simulink model "ASLIPrun2_returnmap"  (R2016a)
settings: Solver=ode45  StartTime=0.0  StopTime=250  MaxStep=1e-3  RelTol=1e-4  AbsTol=1e-6
values from neighbouring files (symbols this model uses):
  a0 = 67*pi/180    (= 1.16937059884)    [ASLIPrun_params2.m]
  dt0 = deg2rad(0)    [ASLIPrun_params2.m]
  dx0 = 5.00    (= 5)    [ASLIPrun_params2.m]
  dy0 = 0    [ASLIPrun_params2.m]
  g = 9.81    [ASLIPrun_params2.m]
  J = 4.58    [ASLIPrun_params2.m]
  k = 20000    [ASLIPrun_params2.m]
  kt = 100    [ASLIPrun_params2.m]
  L = 0.1    [ASLIPrun_params2.m]    (also in AnimSMR2.m = sqrt( (u(4)-u(9))^2 + (u(5)-u(10))^2 ))
  l0 = 1    [ASLIPrun_params2.m]
  m = 80    [ASLIPrun_params2.m]
  model = 1    [ASLIPrun_params2.m]
  r0 = sqrt(xr0^2 + yr0^2)    [ASLIPrun_params2.m]
  rp = 0.005    [ASLIPrun_params2.m]
  t0 = 70*pi/180    (= 1.2217304764)    [ASLIPrun_params2.m]
  x0 = 0*(-l0 + L*cos(t0))    [ASLIPrun_params2.m]    (also in AnimSMR2.m = [])
  xr0 = -l0*cos(a0) + L*cos(t0)    [ASLIPrun_params2.m]
  y0 = 1.065    [ASLIPrun_params2.m]
  yr0 = l0*sin(a0) + L*sin(t0)    [ASLIPrun_params2.m]
libraries: simulink_extras x1
settings Model: Creator=hgeyer  LastModifiedBy=Joe
settings DataIOCC: SaveFormat=Array  SignalLoggingSaveFormat=ModelDataLogs
settings OptimizationCC: ExpressionDepthLimit=2147483647
settings DebuggingCC: UnderspecifiedInitializationDetection=Classic  MergeDetectMultiDrivingBlocksExec=none  SolverPrmCheckMsg=warning  FcnCallInpInsideContextMsg=EnableAllAsWarning  StateNameClashWarn=warning
settings HardwareCC: ProdBitPerPointer=32  ProdLargestAtomicFloat=None  ProdIntDivRoundTo=Undefined  ProdEndianess=Unspecified  ProdWordSize=32  ProdHWDeviceType=32-bit Generic
settings ModelReferenceCC: PropagateSignalLabelsOutOfModel=off
settings ConfigComp: CovModelRefEnable=Off

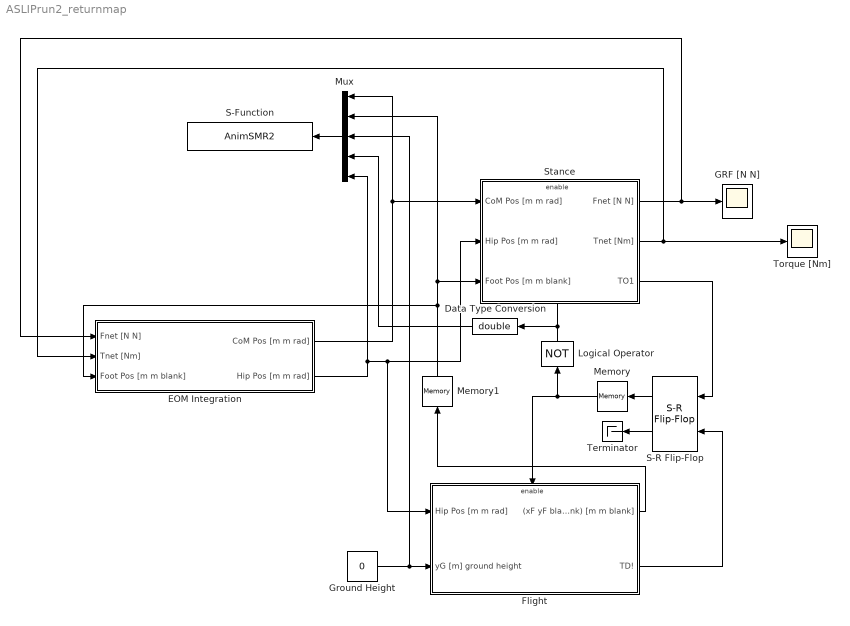
== system ASLIPrun2_returnmap ==
  Data Type Conversion : DataTypeConversion  OutDataTypeStr=double
  EOM Integration : Subsystem
  Flight : Subsystem
  GRF [N N] : Scope
  Ground Height : Constant  Value=0
  Logical Operator : Logic  Operator=NOT  AllPortsSameDT=off  OutDataTypeStr=boolean
  Memory : Memory  X0=1
  Memory1 : Memory  X0="[(x0 - xr0) (y0 - yr0)  0]"
  Mux : Mux  Inputs=5
  S-Function : S-Function  FunctionName=AnimSMR2  Parameters=0.005  SFunctionDeploymentMode=off  EnableBusSupport=off
  S-R Flip-Flop : simulink_extras/Flip Flops/S-R Flip-Flop  initial_condition=1
  Stance : Subsystem
  Terminator : Terminator
  Torque [Nm] : Scope
  wires:
  EOM Integration/1(CoM Pos [m m rad]) -> Stance/1("CoM Pos [m m rad] "), Mux/1
  Stance/3(TO1) -> S-R Flip-Flop/1
  S-R Flip-Flop/1 -> Memory/1
  Logical Operator/1 -> Data Type Conversion/1, Stance/Enable
  Memory/1 -> Logical Operator/1, Flight/Enable
  Flight/2(TD!) -> S-R Flip-Flop/2
  Stance/1(Fnet [N N]) -> EOM Integration/1(Fnet [N N]), GRF [N N]/1
  Flight/1((xF yF blank) [m m blank]) -> Memory1/1
  Memory1/1 -> EOM Integration/3(Foot Pos [m m blank]), Mux/2, Stance/3(Foot Pos [m m blank])
  Mux/1 -> S-Function/1
  S-R Flip-Flop/2 -> Terminator/1
  Ground Height/1 -> Mux/3, Flight/2(yG [m] ground height)
  Data Type Conversion/1 -> Mux/4
  EOM Integration/2(Hip Pos [m m rad]) -> Mux/5, Stance/2(Hip Pos [m m rad]), Flight/1(Hip Pos [m m rad])
  Stance/2(Tnet [Nm]) -> Torque [Nm]/1, EOM Integration/2(Tnet [Nm])

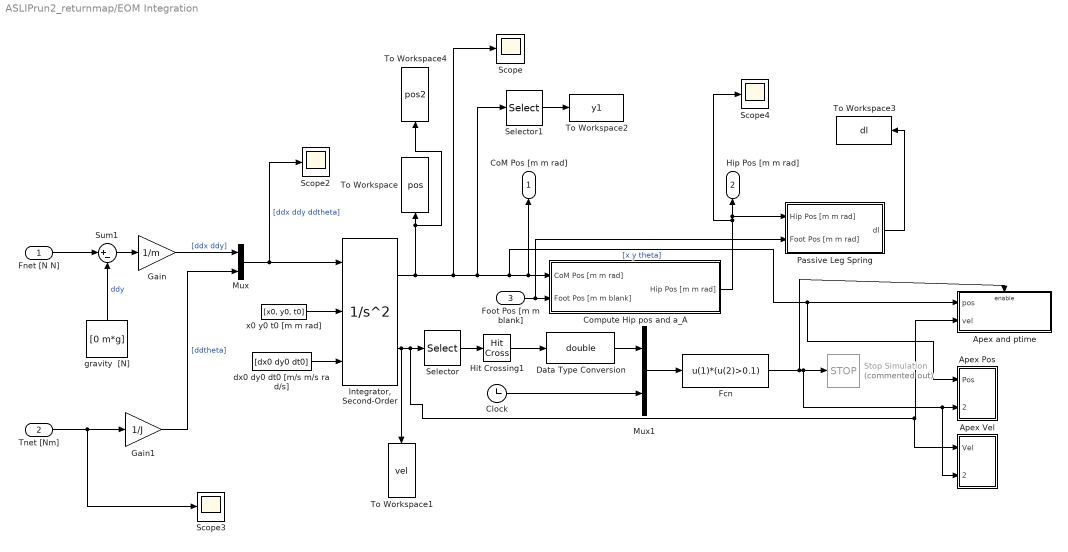
== system ASLIPrun2_returnmap/EOM Integration ==
  Fnet [N N] : Inport
  Tnet [Nm] : Inport  Port=2
  Foot Pos [m m blank] : Inport  Port=3
  Apex Pos : Subsystem
  Apex Vel : Subsystem
  Apex and ptime : Subsystem  TreatAsAtomicUnit=on
  Clock : Clock
  Compute Hip pos and a_A : Subsystem
  Data Type Conversion : DataTypeConversion  OutDataTypeStr=double
  Fcn : Fcn  Expr=u(1)*(u(2)>0.1)
  Gain : Gain  Gain=1/m
  Gain1 : Gain  Gain=1/J
  Hit Crossing1 : HitCross  HitCrossingDirection=falling
  "Integrator, Second-Order" : SecondOrderIntegrator  ICSourceX=external  ICSourceDXDT=external
  Mux : Mux  Inputs=2
  Mux1 : Mux  Inputs=2
  Passive Leg Spring : Subsystem
  Scope{,2..4} (4 alike) : Scope
  Selector : Selector  InputPortWidth=3  IndexOptions=Index vector (dialog)  Indices=[2]  OutputSizes=1
  Selector1 : Selector  InputPortWidth=3  IndexOptions=Index vector (dialog)  Indices=[2]  OutputSizes=1
  Stop Simulation : Stop  Commented=on
  Sum1 : Sum  Inputs=|+-
  To Workspace : ToWorkspace  VariableName=pos  SampleTime=-1
  To Workspace1 : ToWorkspace  VariableName=vel  SampleTime=-1
  To Workspace2 : ToWorkspace  VariableName=y1  SaveFormat=Structure With Time  SampleTime=-1
  To Workspace3 : ToWorkspace  VariableName=dl  SampleTime=-1
  To Workspace4 : ToWorkspace  VariableName=pos2  SaveFormat=Timeseries  SampleTime=-1
  dx0 dy0 dt0 [m/s m/s ra d/s] : Constant  Value=[dx0 dy0 dt0]
  gravity  [N] : Constant  Value=[0 m*g]
  x0 y0 t0 [m m rad] : Constant  Value=[x0, y0, t0]
  CoM Pos [m m rad] : Outport
  Hip Pos [m m rad] : Outport  Port=2
  wires:
  Sum1/1 -> Gain/1
  gravity  [N]/1 -> Sum1/2  "ddy"
  x0 y0 t0 [m m rad]/1 -> "Integrator, Second-Order"/2
  Gain/1 -> Mux/1  "[ddx ddy]"
  Fnet [N N]/1 -> Sum1/1
  dx0 dy0 dt0 [m/s m/s ra d/s]/1 -> "Integrator, Second-Order"/3
  Mux/1 -> Scope2/1, "Integrator, Second-Order"/1  "[ddx ddy ddtheta]"
  Gain1/1 -> Mux/2  "[ddtheta]"
  Tnet [Nm]/1 -> Scope3/1, Gain1/1
  "Integrator, Second-Order"/1 -> Scope/1, Selector1/1, Apex Pos/1(Pos), Apex and ptime/1(pos), Compute Hip pos and a_A/1(CoM Pos [m m rad]), CoM Pos [m m rad]/1, To Workspace4/1, To Workspace/1  "[x y theta]"
  Foot Pos [m m blank]/1 -> Passive Leg Spring/2(Foot Pos [m m rad]), Compute Hip pos and a_A/2(Foot Pos [m m blank])
  Compute Hip pos and a_A/1(Hip Pos [m m rad]) -> Scope4/1, Hip Pos [m m rad]/1, Passive Leg Spring/1(Hip Pos [m m rad])
  Hit Crossing1/1 -> Data Type Conversion/1
  Clock/1 -> Mux1/2
  Mux1/1 -> Fcn/1
  Selector1/1 -> To Workspace2/1
  Passive Leg Spring/1(dl) -> To Workspace3/1
  Selector/1 -> Hit Crossing1/1
  Data Type Conversion/1 -> Mux1/1
  Fcn/1 -> Apex Vel/2(Apex Event), Apex Pos/2(Apex Event), Stop Simulation/1, Apex and ptime/Enable
  "Integrator, Second-Order"/2 -> Apex Vel/1(Vel), Apex and ptime/2(vel), Selector/1, To Workspace1/1

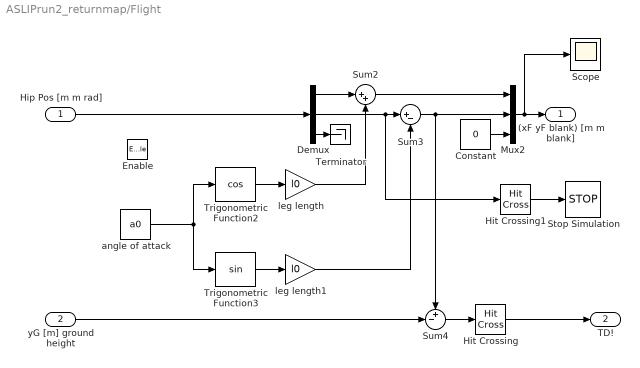
== system ASLIPrun2_returnmap/Flight ==
  Hip Pos [m m rad] : Inport
  yG [m] ground height : Inport  Port=2
  Enable : EnablePort  StatesWhenEnabling=reset
  Constant : Constant  Value=0
  Demux : Demux  Outputs=3
  Hit Crossing : HitCross  HitCrossingDirection=falling
  Hit Crossing1 : HitCross  HitCrossingDirection=falling
  Mux2 : Mux  Inputs=3
  Scope : Scope
  Stop Simulation : Stop
  Sum2 : Sum  Inputs=|++
  Sum3 : Sum  Inputs=|+-
  Sum4 : Sum  Inputs=+-|
  Terminator : Terminator
  Trigonometric Function2 : Trigonometry  Operator=cos
  Trigonometric Function3 : Trigonometry
  angle of attack : Constant  Value=a0
  leg length : Gain  Gain=l0
  leg length1 : Gain  Gain=l0
  (xF yF blank) [m m blank] : Outport  InitialOutput=[0 0 0]
      settings: AttributesFormatString=%<OutputWhenDisabled>
  TD! : Outport  Port=2  OutputWhenDisabled=reset  InitialOutput=0
      settings: AttributesFormatString=%<OutputWhenDisabled>
  wires:
  Hit Crossing/1 -> TD!/1
  Demux/2 -> Hit Crossing1/1, Sum3/1
  Demux/1 -> Sum2/1
  angle of attack/1 -> Trigonometric Function3/1, Trigonometric Function2/1
  Trigonometric Function2/1 -> leg length/1
  Trigonometric Function3/1 -> leg length1/1
  Hip Pos [m m rad]/1 -> Demux/1
  leg length/1 -> Sum2/2
  leg length1/1 -> Sum3/2
  Sum3/1 -> Mux2/2, Sum4/1
  Sum2/1 -> Mux2/1
  Mux2/1 -> Scope/1, (xF yF blank) [m m blank]/1
  yG [m] ground height/1 -> Sum4/2
  Sum4/1 -> Hit Crossing/1
  Constant/1 -> Mux2/3
  Hit Crossing1/1 -> Stop Simulation/1
  Demux/3 -> Terminator/1

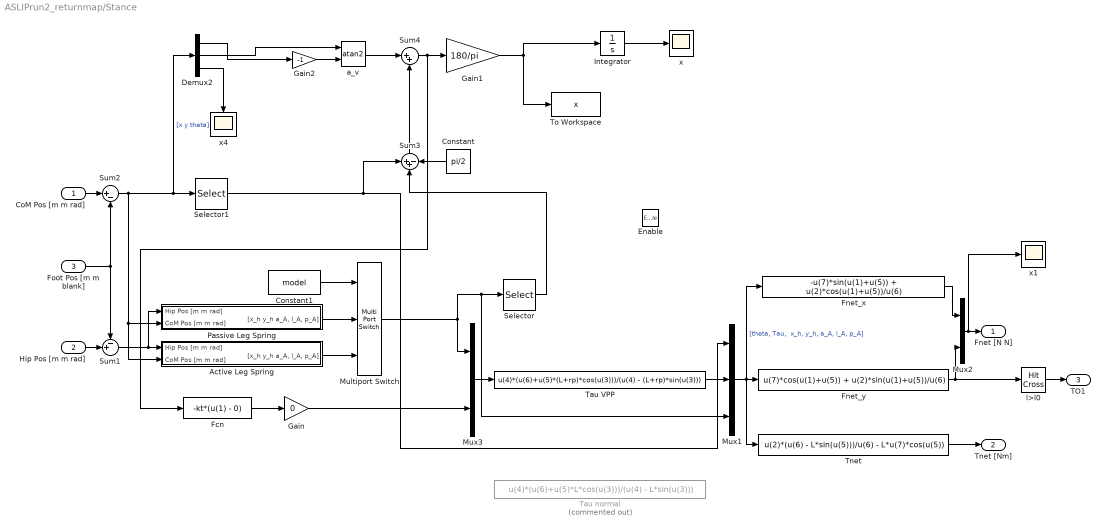
== system ASLIPrun2_returnmap/Stance ==
  "CoM Pos [m m rad] " : Inport
  Hip Pos [m m rad] : Inport  Port=2
  Foot Pos [m m blank] : Inport  Port=3
  Enable : EnablePort  StatesWhenEnabling=reset
  Active Leg Spring : Subsystem
  Constant : Constant  Value=pi/2
  Constant1 : Constant  Value=model
  Demux2 : Demux  Outputs=3
  Fcn : Fcn  Expr=-kt*(u(1) - 0)
  Fnet_x : Fcn  Expr=-u(7)*sin(u(1)+u(5)) + u(2)*cos(u(1)+u(5))/u(6)
  Fnet_y : Fcn  Expr=u(7)*cos(u(1)+u(5)) + u(2)*sin(u(1)+u(5))/u(6)
  Gain : Gain  Gain=0
  Gain1 : Gain  Gain=180/pi
  Gain2 : Gain  Gain=-1
  Integrator : Integrator
  Multiport Switch : MultiPortSwitch  Inputs=2
  Mux1 : Mux  Inputs=3
  Mux2 : Mux  Inputs=2
  Mux3 : Mux  Inputs=2
  Passive Leg Spring : Subsystem
  Selector : Selector  InputPortWidth=5  IndexOptions=Index vector (dialog)  Indices=[3]  OutputSizes=1
  Selector1 : Selector  InputPortWidth=3  IndexOptions=Index vector (dialog)  Indices=[3]  OutputSizes=1
  Sum1 : Sum  Inputs=-+|
  Sum2 : Sum  Inputs=|+-
  Sum3 : Sum  Inputs=++-
  Sum4 : Sum  Inputs=|++
  Tau VPP : Fcn  Expr=u(4)*(u(6)+u(5)*(L+rp)*cos(u(3)))/(u(4) - (L+rp)*sin(u(3)))
  Tau normal : Fcn  Commented=on  Expr=u(4)*(u(6)+u(5)*L*cos(u(3)))/(u(4) - L*sin(u(3)))
  Tnet : Fcn  Expr=u(2)*(u(6) - L*sin(u(5)))/u(6) - L*u(7)*cos(u(5))
  To Workspace : ToWorkspace  VariableName=x  SaveFormat=Timeseries  SampleTime=-1
  a_v : Trigonometry  Operator=atan2
  l>l0 : HitCross  HitCrossingOffset=l0  HitCrossingDirection=falling
  x : Scope
  x1 : Scope
  x4 : Scope
  Fnet [N N] : Outport  OutputWhenDisabled=reset  InitialOutput=[0,0]
  Tnet [Nm] : Outport  Port=2  OutputWhenDisabled=reset  InitialOutput=[0]
  TO1 : Outport  Port=3  OutputWhenDisabled=reset  InitialOutput=[0]
  wires:
  Tau VPP/1 -> Mux1/2
  Selector1/1 -> Mux1/1, Sum3/1
  Fnet_x/1 -> Mux2/1
  Tnet/1 -> Tnet [Nm]/1
  "CoM Pos [m m rad] "/1 -> Sum2/1
  Sum1/1 -> Passive Leg Spring/1(Hip Pos [m m rad]), Active Leg Spring/1(Hip Pos [m m rad])
  Hip Pos [m m rad]/1 -> Sum1/2
  Mux1/1 -> Tnet/1, Fnet_x/1, Fnet_y/1  "[theta, Tau,  x_h, y_h, a_A, l_A, p_A]"
  Foot Pos [m m blank]/1 -> Sum2/2, Sum1/1
  Sum2/1 -> Active Leg Spring/2(CoM Pos [m m rad]), Passive Leg Spring/2(CoM Pos [m m rad]), Selector1/1, Demux2/1  "[x y theta]"
  Demux2/1 -> Gain2/1
  Demux2/3 -> x4/1
  a_v/1 -> Sum4/1
  Constant/1 -> Sum3/3
  Sum3/1 -> Sum4/2
  Gain2/1 -> a_v/2
  Demux2/2 -> a_v/1
  Gain1/1 -> To Workspace/1, Integrator/1
  Sum4/1 -> Fcn/1, Gain1/1
  Mux2/1 -> x1/1, Fnet [N N]/1
  Fnet_y/1 -> l>l0/1, Mux2/2
  Selector/1 -> Sum3/2
  l>l0/1 -> TO1/1
  Mux3/1 -> Tau VPP/1
  Multiport Switch/1 -> Mux3/1, Mux1/3, Selector/1
  Gain/1 -> Mux3/2
  Fcn/1 -> Gain/1
  Passive Leg Spring/1("[x_h y_h a_A, l_A, p_A]") -> Multiport Switch/2
  Active Leg Spring/1("[x_h y_h a_A, l_A, p_A]") -> Multiport Switch/3
  Constant1/1 -> Multiport Switch/1
  Integrator/1 -> x/1

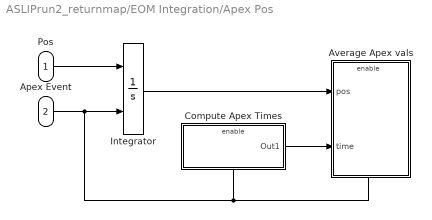
== system ASLIPrun2_returnmap/EOM Integration/Apex Pos ==
  Pos : Inport
  Apex Event : Inport  Port=2
  Average Apex vals : Subsystem  TreatAsAtomicUnit=on
  Compute Apex Times : Subsystem  TreatAsAtomicUnit=on
  Integrator : Integrator  ExternalReset=falling  InitialCondition=[0,0,0]
  wires:
  Integrator/1 -> Average Apex vals/1(pos)
  Compute Apex Times/1(Out1) -> Average Apex vals/2(time)
  Apex Event/1 -> Integrator/2, Average Apex vals/Enable, Compute Apex Times/Enable
  Pos/1 -> Integrator/1

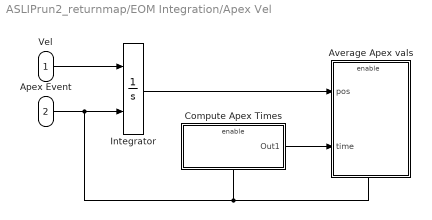
== system ASLIPrun2_returnmap/EOM Integration/Apex Vel ==
  Vel : Inport
  Apex Event : Inport  Port=2
  Average Apex vals : Subsystem  TreatAsAtomicUnit=on
  Compute Apex Times : Subsystem  TreatAsAtomicUnit=on
  Integrator : Integrator  ExternalReset=falling  InitialCondition=[0,0,0]
  wires:
  Vel/1 -> Integrator/1
  Apex Event/1 -> Compute Apex Times/Enable, Average Apex vals/Enable, Integrator/2
  Compute Apex Times/1(Out1) -> Average Apex vals/2(time)
  Integrator/1 -> Average Apex vals/1(pos)

== system ASLIPrun2_returnmap/EOM Integration/Apex and ptime ==
  pos : Inport
  vel : Inport  Port=2
  Enable : EnablePort
  To Workspace1 : ToWorkspace  VariableName=apexvel  SaveFormat=Timeseries  SampleTime=-1
  To Workspace3 : ToWorkspace  VariableName=apexpos  SaveFormat=Timeseries  SampleTime=-1
  wires:
  pos/1 -> To Workspace3/1
  vel/1 -> To Workspace1/1

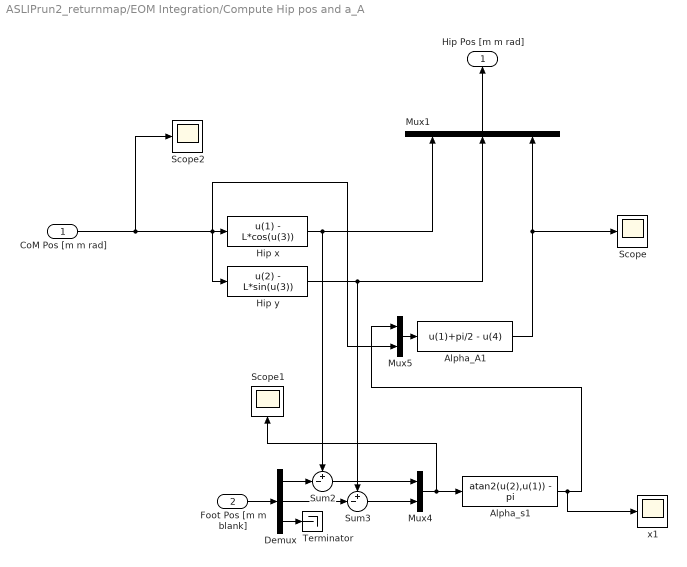
== system ASLIPrun2_returnmap/EOM Integration/Compute Hip pos and a_A ==
  CoM Pos [m m rad] : Inport
  Foot Pos [m m blank] : Inport  Port=2
  Alpha_A1 : Fcn  Expr=u(1)+pi/2 - u(4)
  Alpha_s1 : Fcn  Expr=atan2(u(2),u(1)) - pi
  Demux : Demux  Outputs=3
  Hip x : Fcn  Expr=u(1) - L*cos(u(3))
  Hip y : Fcn  Expr=u(2) - L*sin(u(3))
  Mux1 : Mux  Inputs=3
  Mux4 : Mux  Inputs=2
  Mux5 : Mux  Inputs=2
  Scope : Scope
  Scope1 : Scope
  Scope2 : Scope
  Sum2 : Sum  Inputs=+-|
  Sum3 : Sum  Inputs=+-|
  Terminator : Terminator
  x1 : Scope
  Hip Pos [m m rad] : Outport
  wires:
  CoM Pos [m m rad]/1 -> Scope2/1, Hip x/1, Hip y/1, Mux5/2
  Mux4/1 -> Alpha_s1/1, Scope1/1
  Mux5/1 -> Alpha_A1/1
  Hip x/1 -> Sum2/1, Mux1/1
  Mux1/1 -> Hip Pos [m m rad]/1
  Hip y/1 -> Sum3/1, Mux1/2
  Alpha_s1/1 -> x1/1, Mux5/1
  Demux/2 -> Sum3/2
  Demux/3 -> Terminator/1
  Sum2/1 -> Mux4/1
  Demux/1 -> Sum2/2
  Alpha_A1/1 -> Mux1/3, Scope/1
  Foot Pos [m m blank]/1 -> Demux/1
  Sum3/1 -> Mux4/2

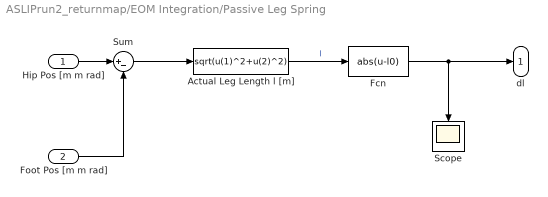
== system ASLIPrun2_returnmap/EOM Integration/Passive Leg Spring ==
  Hip Pos [m m rad] : Inport
  Foot Pos [m m rad] : Inport  Port=2
  Actual Leg Length l [m] : Fcn  Expr=sqrt(u(1)^2+u(2)^2)
  Fcn : Fcn  Expr=abs(u-l0)
  Scope : Scope
  Sum : Sum  Inputs=|+-
  dl : Outport
  wires:
  Actual Leg Length l [m]/1 -> Fcn/1  "l"
  Foot Pos [m m rad]/1 -> Sum/2
  Fcn/1 -> dl/1, Scope/1
  Hip Pos [m m rad]/1 -> Sum/1
  Sum/1 -> Actual Leg Length l [m]/1

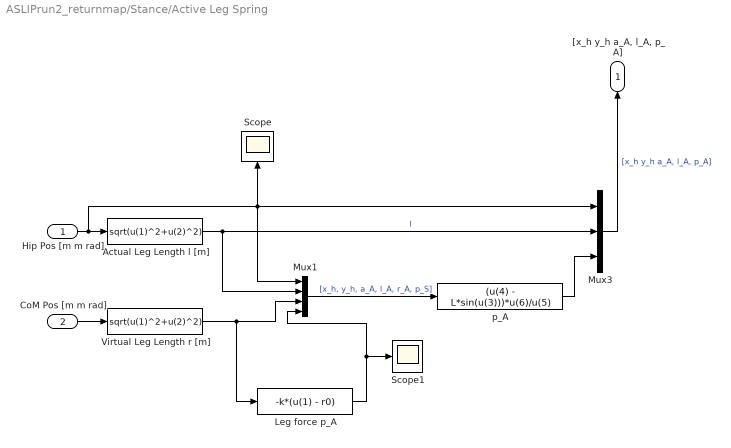
== system ASLIPrun2_returnmap/Stance/Active Leg Spring ==
  Hip Pos [m m rad] : Inport
  CoM Pos [m m rad] : Inport  Port=2
  Actual Leg Length l [m] : Fcn  Expr=sqrt(u(1)^2+u(2)^2)
  Leg force p_A : Fcn  Expr=-k*(u(1) - r0)
  Mux1 : Mux
  Mux3 : Mux  Inputs=3
  Scope : Scope
  Scope1 : Scope
  Virtual Leg Length r [m] : Fcn  Expr=sqrt(u(1)^2+u(2)^2)
  p_A : Fcn  Expr=(u(4) - L*sin(u(3)))*u(6)/u(5)
  "[x_h y_h a_A, l_A, p_A]" : Outport
  wires:
  CoM Pos [m m rad]/1 -> Virtual Leg Length r [m]/1
  p_A/1 -> Mux3/3
  Mux1/1 -> p_A/1  "[x_h, y_h, a_A, l_A, r_A, p_S]"
  Virtual Leg Length r [m]/1 -> Mux1/3, Leg force p_A/1
  Hip Pos [m m rad]/1 -> Mux1/1, Mux3/1, Scope/1, Actual Leg Length l [m]/1
  Actual Leg Length l [m]/1 -> Mux3/2, Mux1/2  "l"
  Mux3/1 -> "[x_h y_h a_A, l_A, p_A]"/1  "[x_h y_h a_A, l_A, p_A]"
  Leg force p_A/1 -> Scope1/1, Mux1/4

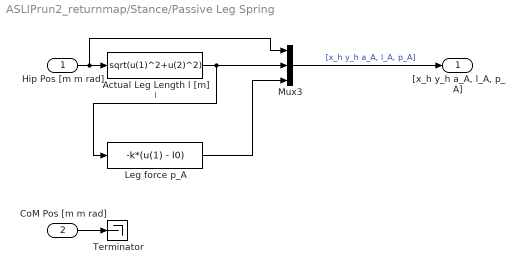
== system ASLIPrun2_returnmap/Stance/Passive Leg Spring ==
  Hip Pos [m m rad] : Inport
  CoM Pos [m m rad] : Inport  Port=2
  Actual Leg Length l [m] : Fcn  Expr=sqrt(u(1)^2+u(2)^2)
  Leg force p_A : Fcn  Expr=-k*(u(1) - l0)
  Mux3 : Mux  Inputs=3
  Terminator : Terminator
  "[x_h y_h a_A, l_A, p_A]" : Outport
  wires:
  Mux3/1 -> "[x_h y_h a_A, l_A, p_A]"/1  "[x_h y_h a_A, l_A, p_A]"
  Actual Leg Length l [m]/1 -> Leg force p_A/1, Mux3/2  "l"
  Leg force p_A/1 -> Mux3/3
  Hip Pos [m m rad]/1 -> Actual Leg Length l [m]/1, Mux3/1
  CoM Pos [m m rad]/1 -> Terminator/1

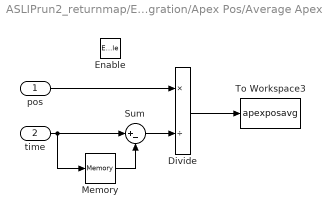
== system ASLIPrun2_returnmap/EOM Integration/Apex Pos/Average Apex vals ==
  pos : Inport
  time : Inport  Port=2
  Enable : EnablePort
  Divide : Product  Inputs=*/
  Memory : Memory
  Sum : Sum  Inputs=|+-
  To Workspace3 : ToWorkspace  VariableName=apexposavg  SaveFormat=Timeseries  SampleTime=-1
  wires:
  pos/1 -> Divide/1
  time/1 -> Memory/1, Sum/1
  Memory/1 -> Sum/2
  Divide/1 -> To Workspace3/1
  Sum/1 -> Divide/2

== system ASLIPrun2_returnmap/EOM Integration/Apex Pos/Compute Apex Times ==
  Enable : EnablePort
  Clock : Clock
  Scope : Scope
  Out1 : Outport  OutputWhenDisabled=reset  InitialOutput=0
  wires:
  Clock/1 -> Out1/1, Scope/1

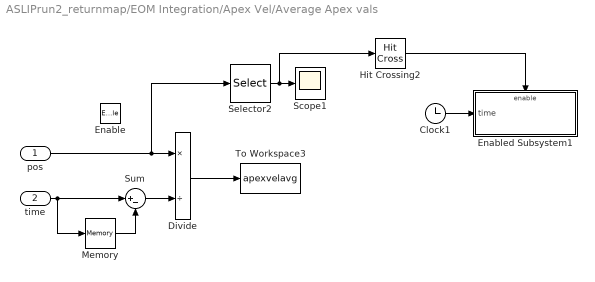
== system ASLIPrun2_returnmap/EOM Integration/Apex Vel/Average Apex vals ==
  pos : Inport
  time : Inport  Port=2
  Enable : EnablePort
  Clock1 : Clock
  Divide : Product  Inputs=*/
  Enabled Subsystem1 : Subsystem  TreatAsAtomicUnit=on
  Hit Crossing2 : HitCross  HitCrossingDirection=falling
  Memory : Memory
  Scope1 : Scope
  Selector2 : Selector  InputPortWidth=3  IndexOptions=Index vector (dialog)  Indices=[3]  OutputSizes=1
  Sum : Sum  Inputs=|+-
  To Workspace3 : ToWorkspace  VariableName=apexvelavg  SaveFormat=Timeseries  SampleTime=-1
  wires:
  Sum/1 -> Divide/2
  Divide/1 -> To Workspace3/1
  Memory/1 -> Sum/2
  time/1 -> Sum/1, Memory/1
  pos/1 -> Selector2/1, Divide/1
  Hit Crossing2/1 -> Enabled Subsystem1/Enable
  Clock1/1 -> Enabled Subsystem1/1(time)
  Selector2/1 -> Hit Crossing2/1, Scope1/1

== system ASLIPrun2_returnmap/EOM Integration/Apex Vel/Compute Apex Times ==
  Enable : EnablePort
  Clock : Clock
  Scope : Scope
  Out1 : Outport  OutputWhenDisabled=reset  InitialOutput=0
  wires:
  Clock/1 -> Scope/1, Out1/1

== system ASLIPrun2_returnmap/EOM Integration/Apex Vel/Average Apex vals/Enabled Subsystem1 ==
  time : Inport
  Enable : EnablePort
  To Workspace3 : ToWorkspace  VariableName=ptime  SampleTime=-1
  wires:
  time/1 -> To Workspace3/1
